simulink model "mod_bio_oxygen"  (R2017a)
settings: Solver=ode45  StartTime=0.0  StopTime=10.0  RelTol=1e-3  EnableMultiTasking=on
settings Model: Creator=Tanay  LastModifiedBy=pum
settings DataIOCC: LimitDataPoints=on  SaveFormat=Array
settings OptimizationCC: LifeSpan=inf
settings DebuggingCC: SolverPrmCheckMsg=warning  SFUnexpectedBacktrackingDiag=warning  SFNoUnconditionalDefaultTransitionDiag=warning  SFExecutionAtInitializationDiag=none
settings HardwareCC: ProdBitPerPointer=32  ProdBitPerSizeT=32  ProdBitPerPtrDiffT=32  ProdLargestAtomicFloat=None  ProdIntDivRoundTo=Undefined  ProdEndianess=Unspecified  ProdWordSize=32  ProdHWDeviceType=32-bit Generic
settings ModelReferenceCC: PropagateSignalLabelsOutOfModel=off
settings GRTTargetCC: TargetLangStandard=C89/C90 (ANSI)  GeneratePreprocessorConditionals=Disable all
settings ConfigComp: CovMetricSettings=dw  CovHtmlReporting=on  CovSaveCumulativeToWorkspaceVar=on  CovSaveSingleToWorkspaceVar=on  CovExternalEMLEnable=off  CovSFcnEnable=off

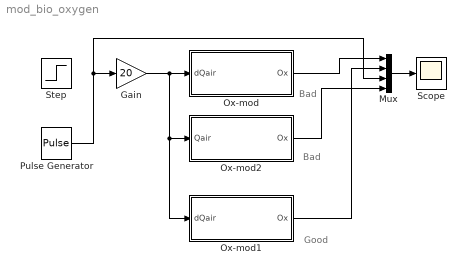
== system mod_bio_oxygen ==
  note: Good
  note: Bad
  note: Bad
  Gain : Gain  Gain=20
  Mux : Mux
  Ox-mod : Subsystem  mask{cx_max=10, alpha=1, beta=1}
      mask prompts: cx_max "Oxygen contents"; alpha "Liquefication speed"; beta "Aeration coef."
  Ox-mod1 : Subsystem  mask{ox_max=10, ox_min=2, alpha=0.5, beta=2}
      mask prompts: ox_max "Maximum"; ox_min "Minimum"; alpha "Coef. aeration"; beta "Coef. de-aeration"
  Ox-mod2 : Subsystem  mask{ox_max=10, ox_min=0.1, alpha=0.5}
      mask prompts: ox_max "Maximum"; ox_min "Minimum"; alpha "Coef. transformation"
  Pulse Generator : DiscretePulseGenerator  PulseType=Time based  Period=5  PulseWidth=50
  Scope : Scope
  Step : Step  SampleTime=0
  wires:
  Ox-mod/1(Ox) -> Mux/1
  Pulse Generator/1 -> Mux/3, Gain/1
  Gain/1 -> Ox-mod2/1(Qair), Ox-mod1/1(dQair), Ox-mod/1(dQair)
  Mux/1 -> Scope/1
  Ox-mod1/1(Ox) -> Mux/2
  Ox-mod2/1(Ox) -> Mux/4

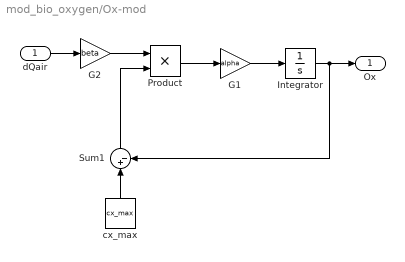
== system mod_bio_oxygen/Ox-mod ==
  dQair : Inport
  G1 : Gain  Gain=alpha
  G2 : Gain  Gain=beta
  Integrator : Integrator
  Product : Product
  Sum1 : Sum  Inputs=|+-
  cx_max : Constant  Value=cx_max
  Ox : Outport
  wires:
  Sum1/1 -> Product/2
  cx_max/1 -> Sum1/1
  dQair/1 -> G2/1
  Product/1 -> G1/1
  Integrator/1 -> Sum1/2, Ox/1
  G1/1 -> Integrator/1
  G2/1 -> Product/1

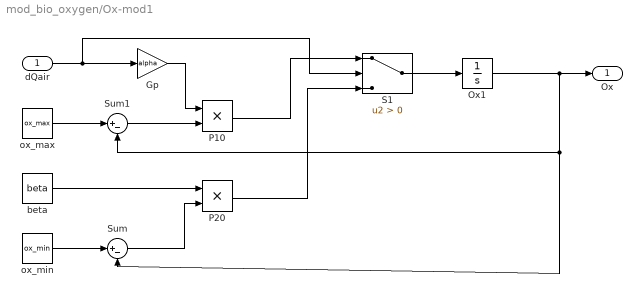
== system mod_bio_oxygen/Ox-mod1 ==
  dQair : Inport
  Gp : Gain  Gain=alpha
  Ox1 : Integrator
  P10 : Product
  P20 : Product
  S1 : Switch  Criteria=u2 > Threshold
  Sum : Sum  Inputs=|+-
  Sum1 : Sum  Inputs=|+-
  beta : Constant  Value=beta
  ox_max : Constant  Value=ox_max
  ox_min : Constant  Value=ox_min
  Ox : Outport
  wires:
  Ox1/1 -> Sum/2, Sum1/2, Ox/1
  ox_max/1 -> Sum1/1
  ox_min/1 -> Sum/1
  S1/1 -> Ox1/1
  dQair/1 -> Gp/1, S1/2
  Sum1/1 -> P10/2
  P10/1 -> S1/1
  Gp/1 -> P10/1
  Sum/1 -> P20/2
  beta/1 -> P20/1
  P20/1 -> S1/3

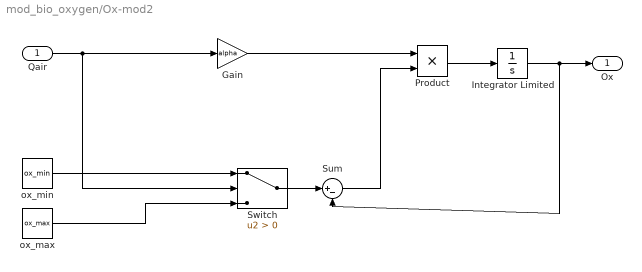
== system mod_bio_oxygen/Ox-mod2 ==
  Qair : Inport
  Gain : Gain  Gain=alpha
  Integrator Limited : Integrator  LimitOutput=on  UpperSaturationLimit=ox_max  LowerSaturationLimit=0
  Product : Product
  Sum : Sum  Inputs=|+-
  Switch : Switch  Criteria=u2 > Threshold
  ox_max : Constant  Value=ox_max
  ox_min : Constant  Value=ox_min
  Ox : Outport
  wires:
  Qair/1 -> Switch/2, Gain/1
  Integrator Limited/1 -> Ox/1, Sum/2
  ox_max/1 -> Switch/3
  ox_min/1 -> Switch/1
  Switch/1 -> Sum/1
  Sum/1 -> Product/2
  Product/1 -> Integrator Limited/1
  Gain/1 -> Product/1
